simulink model "untitled"  (R2018b)
settings: Solver=FixedStepAuto  StartTime=0.0  StopTime=50  FixedStep=0.001  RelTol=1e-3
settings Model: Creator=giga4  LastModifiedBy=giga4

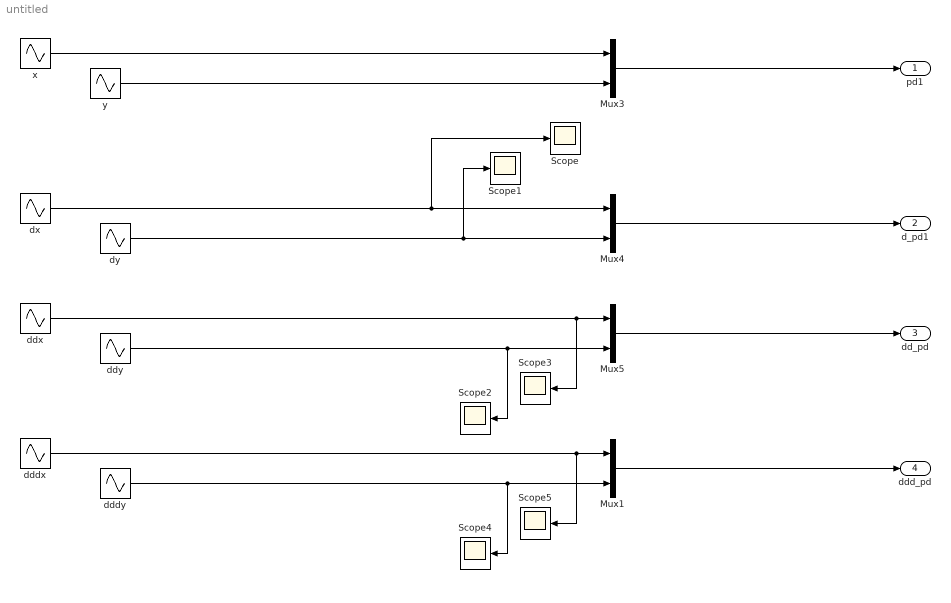
== system untitled ==
  Mux{1,3..5} (4 alike) : Mux  Inputs=2
  Scope{,1..5} (6 alike) : Scope
  dddx : Sin  Amplitude=10  SampleTime=0
  dddy : Sin  Amplitude=-10  Phase=pi/2  SampleTime=0
  ddx : Sin  Amplitude=-10  Phase=pi/2  SampleTime=0
  ddy : Sin  Amplitude=-10  SampleTime=0
  dx : Sin  Amplitude=-10  SampleTime=0
  dy : Sin  Amplitude=10  Phase=pi/2  SampleTime=0
  x : Sin  Amplitude=10  Phase=pi/2  SampleTime=0
  y : Sin  Amplitude=10  SampleTime=0
  pd1 : Outport
  d_pd1 : Outport  Port=2
  dd_pd : Outport  Port=3
  ddd_pd : Outport  Port=4
  wires:
  Mux4/1 -> d_pd1/1
  ddx/1 -> Scope3/1, Mux5/1
  Mux5/1 -> dd_pd/1
  dy/1 -> Scope1/1, Mux4/2
  dx/1 -> Scope/1, Mux4/1
  ddy/1 -> Scope2/1, Mux5/2
  Mux3/1 -> pd1/1
  y/1 -> Mux3/2
  x/1 -> Mux3/1
  dddx/1 -> Scope5/1, Mux1/1
  Mux1/1 -> ddd_pd/1
  dddy/1 -> Scope4/1, Mux1/2
